simulink library "PortLib"  (Simulink 7.6)
settings: Solver=ode45  StartTime=0.0  StopTime=10.0  RelTol=1e-3
libraries: orocos_taskcontext x31, simulink x22
settings Model: Creator=Haus  LastModifiedBy=sendobry

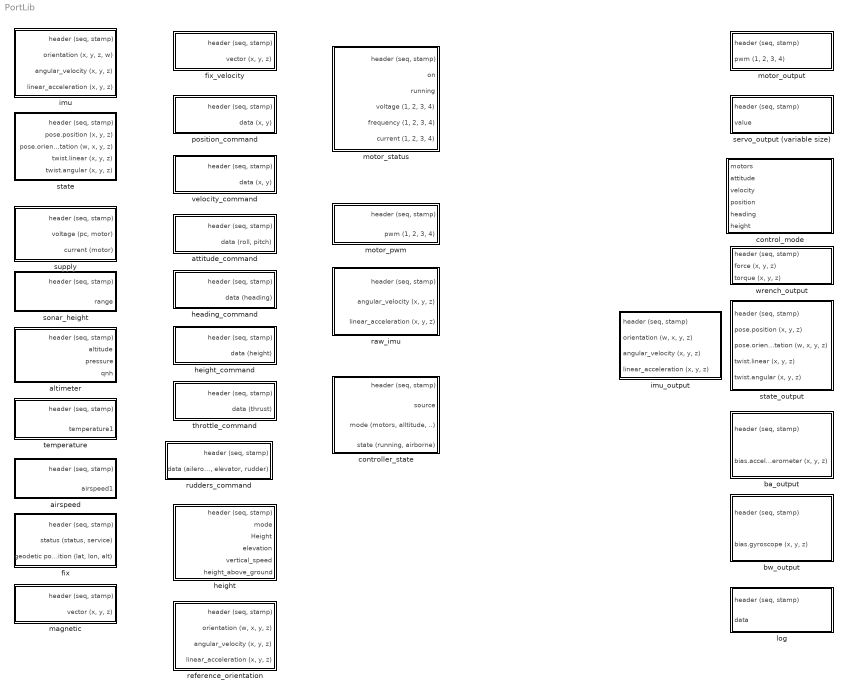
== system PortLib ==
  airspeed : Subsystem
  altimeter : Subsystem
  attitude_command : Subsystem
  ba_output : Subsystem
  bw_output : Subsystem
  control_mode : Subsystem
  controller_state : Subsystem
  fix : Subsystem
  fix_velocity : Subsystem
  heading_command : Subsystem
  height : Subsystem
  height_command : Subsystem
  imu : Subsystem
  imu_output : Subsystem
  log : Subsystem
  magnetic : Subsystem
  motor_output : Subsystem
  motor_pwm : Subsystem
  motor_status : Subsystem
  position_command : Subsystem
  raw_imu : Subsystem
  reference_orientation : Subsystem
  rudders_command : Subsystem
  servo_output (variable size) : Subsystem
  sonar_height : Subsystem
  state : Subsystem
  state_output : Subsystem
  supply : Subsystem
  temperature : Subsystem
  throttle_command : Subsystem
  velocity_command : Subsystem  AncestorBlock=PortLib/PositionXYCommand
  wrench_output : Subsystem

== system PortLib/airspeed ==
  Selector : Selector  IndexMode=Zero-based  InputPortWidth=3  IndexOptions=Index vector (dialog)  Indices=[0 1]  OutputSizes=1
  Selector1 : Selector  IndexMode=Zero-based  InputPortWidth=3  IndexOptions=Index vector (dialog)  Indices=[2]  OutputSizes=1
  airspeed : orocos_taskcontext/InputPort<array>  dpdesc=Port's Description  dpvalue=zeros(1,3)
      settings: AttributesFormatString=Value=%<dpvalue>
  "header (seq, stamp)" : Outport
  airspeed1 : Outport  Port=2
  wires:
  Selector/1 -> "header (seq, stamp)"/1
  airspeed/1 -> Selector1/1, Selector/1
  Selector1/1 -> airspeed1/1

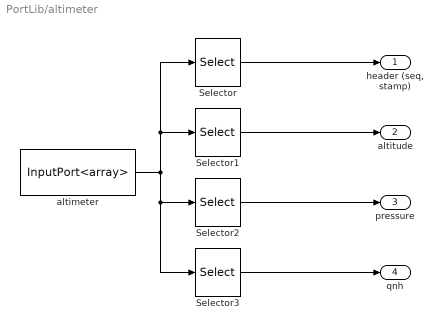
== system PortLib/altimeter ==
  Selector : Selector  IndexMode=Zero-based  InputPortWidth=5  IndexOptions=Index vector (dialog)  Indices=[0 1]  OutputSizes=1
  Selector1 : Selector  IndexMode=Zero-based  InputPortWidth=5  IndexOptions=Index vector (dialog)  Indices=[2]  OutputSizes=1
  Selector2 : Selector  IndexMode=Zero-based  InputPortWidth=5  IndexOptions=Index vector (dialog)  Indices=[3]  OutputSizes=1
  Selector3 : Selector  IndexMode=Zero-based  InputPortWidth=5  IndexOptions=Index vector (dialog)  Indices=[4]  OutputSizes=1
  altimeter : orocos_taskcontext/InputPort<array>  dpdesc=Port's Description  dpvalue=zeros(1,5)
      settings: AttributesFormatString=Value=%<dpvalue>
  "header (seq, stamp)" : Outport
  altitude : Outport  Port=2
  pressure : Outport  Port=3
  qnh : Outport  Port=4
  wires:
  Selector/1 -> "header (seq, stamp)"/1
  altimeter/1 -> Selector1/1, Selector/1, Selector2/1, Selector3/1
  Selector2/1 -> pressure/1
  Selector1/1 -> altitude/1
  Selector3/1 -> qnh/1

== system PortLib/attitude_command ==
  Selector : Selector  IndexMode=Zero-based  InputPortWidth=4  IndexOptions=Index vector (dialog)  Indices=[0 1]  OutputSizes=1
  Selector1 : Selector  IndexMode=Zero-based  InputPortWidth=4  IndexOptions=Index vector (dialog)  Indices=[2 3]  OutputSizes=1
  attitude_command : orocos_taskcontext/InputPort<array>  dpdesc=Port's Description  dpvalue=zeros(1,4)
      settings: AttributesFormatString=Value=%<dpvalue>
  "header (seq, stamp)" : Outport
  "data (roll, pitch)" : Outport  Port=2
  wires:
  Selector/1 -> "header (seq, stamp)"/1
  attitude_command/1 -> Selector1/1, Selector/1
  Selector1/1 -> "data (roll, pitch)"/1

== system PortLib/ba_output ==
  "header (seq, stamp)" : Inport
  "bias.accelerometer (x, y, z)" : Inport  Port=2
  Mux1 : Mux  Inputs=2
  linear_acceleration_bias : orocos_taskcontext/OutputPort<array>  dpdesc=Port's Description  dpvalue=zeros(1,5)
      settings: AttributesFormatString=Value=%<dpvalue>
  wires:
  "header (seq, stamp)"/1 -> Mux1/1
  "bias.accelerometer (x, y, z)"/1 -> Mux1/2
  Mux1/1 -> linear_acceleration_bias/1

== system PortLib/bw_output ==
  "header (seq, stamp)" : Inport
  "bias.gyroscope (x, y, z)" : Inport  Port=2
  Mux1 : Mux  Inputs=2
  angular_velocity_bias : orocos_taskcontext/OutputPort<array>  dpdesc=Port's Description  dpvalue=zeros(1,5)
      settings: AttributesFormatString=Value=%<dpvalue>
  wires:
  Mux1/1 -> angular_velocity_bias/1
  "bias.gyroscope (x, y, z)"/1 -> Mux1/2
  "header (seq, stamp)"/1 -> Mux1/1

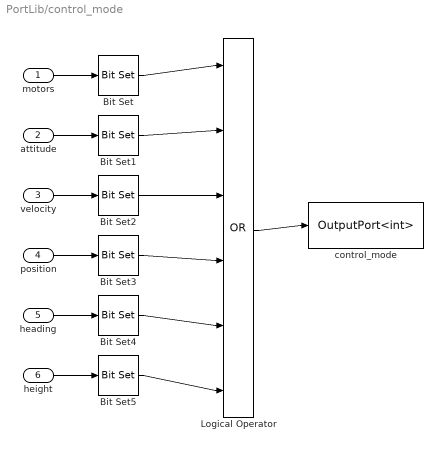
== system PortLib/control_mode ==
  motors : Inport
  attitude : Inport  Port=2
  velocity : Inport  Port=3
  position : Inport  Port=4
  heading : Inport  Port=5
  height : Inport  Port=6
  Bit Set : simulink/Logic and Bit Operations/Bit Set  iBit=0
  Bit Set1 : simulink/Logic and Bit Operations/Bit Set  iBit=1
  Bit Set2 : simulink/Logic and Bit Operations/Bit Set  iBit=2
  Bit Set3 : simulink/Logic and Bit Operations/Bit Set  iBit=3
  Bit Set4 : simulink/Logic and Bit Operations/Bit Set  iBit=4
  Bit Set5 : simulink/Logic and Bit Operations/Bit Set  iBit=5
  Logical Operator : Logic  Operator=OR  Inputs=6  AllPortsSameDT=off  OutDataTypeStr=boolean
  control_mode : orocos_taskcontext/OutputPort<int>  dpdesc=Port's Description  dpvalue=int32(0)
      settings: AttributesFormatString=Value=%<dpvalue>
  wires:
  Logical Operator/1 -> control_mode/1
  motors/1 -> Bit Set/1
  Bit Set/1 -> Logical Operator/1
  Bit Set1/1 -> Logical Operator/2
  Bit Set2/1 -> Logical Operator/3
  Bit Set3/1 -> Logical Operator/4
  Bit Set4/1 -> Logical Operator/5
  heading/1 -> Bit Set4/1
  position/1 -> Bit Set3/1
  velocity/1 -> Bit Set2/1
  attitude/1 -> Bit Set1/1
  height/1 -> Bit Set5/1
  Bit Set5/1 -> Logical Operator/6

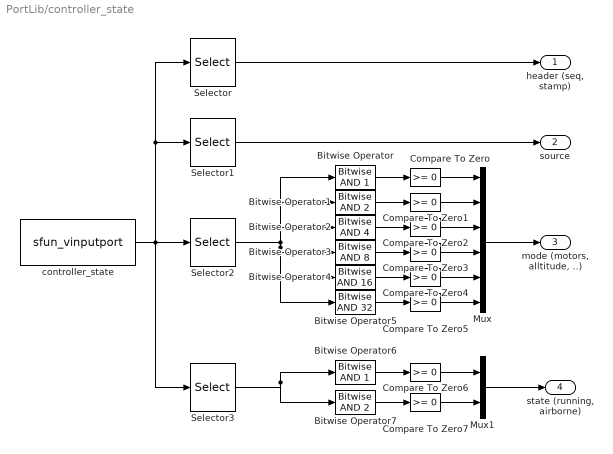
== system PortLib/controller_state ==
  Bitwise Operator : simulink/Logic and Bit Operations/Bitwise Operator  logicop=AND  UseBitMask=on  BitMask=1  BitMaskRealWorld=Stored Integer
  Bitwise Operator1 : simulink/Logic and Bit Operations/Bitwise Operator  logicop=AND  UseBitMask=on  BitMask=2  BitMaskRealWorld=Stored Integer
  Bitwise Operator2 : simulink/Logic and Bit Operations/Bitwise Operator  logicop=AND  UseBitMask=on  BitMask=4  BitMaskRealWorld=Stored Integer
  Bitwise Operator3 : simulink/Logic and Bit Operations/Bitwise Operator  logicop=AND  UseBitMask=on  BitMask=8  BitMaskRealWorld=Stored Integer
  Bitwise Operator4 : simulink/Logic and Bit Operations/Bitwise Operator  logicop=AND  UseBitMask=on  BitMask=16  BitMaskRealWorld=Stored Integer
  Bitwise Operator5 : simulink/Logic and Bit Operations/Bitwise Operator  logicop=AND  UseBitMask=on  BitMask=32  BitMaskRealWorld=Stored Integer
  Bitwise Operator6 : simulink/Logic and Bit Operations/Bitwise Operator  logicop=AND  UseBitMask=on  BitMask=1  BitMaskRealWorld=Stored Integer
  Bitwise Operator7 : simulink/Logic and Bit Operations/Bitwise Operator  logicop=AND  UseBitMask=on  BitMask=2  BitMaskRealWorld=Stored Integer
  Compare To Zero{,1..7} (8 alike) : simulink/Logic and Bit Operations/Compare To Zero  relop=>=  OutDataTypeStr=boolean
  Mux : Mux  Inputs=6
  Mux1 : Mux  Inputs=2
  Selector : Selector  IndexMode=Zero-based  InputPortWidth=5  IndexOptions=Index vector (dialog)  Indices=[0 1]  OutputSizes=1
  Selector1 : Selector  IndexMode=Zero-based  InputPortWidth=5  IndexOptions=Index vector (dialog)  Indices=2  OutputSizes=1
  Selector2 : Selector  IndexMode=Zero-based  InputPortWidth=5  IndexOptions=Index vector (dialog)  Indices=3  OutputSizes=1
  Selector3 : Selector  IndexMode=Zero-based  InputPortWidth=5  IndexOptions=Index vector (dialog)  Indices=4  OutputSizes=1
  controller_state : S-Function  FunctionName=sfun_vinputport  Parameters=dpdesc,dpvalue  EnableBusSupport=off  mask(DataPort<array>){dpdesc=Port's Description, dpvalue=zeros(1,5)}
      mask prompts: dpdesc "Description"; dpvalue "Initial Value (array)"
      mask help: A TaskContext's Vector DataPort holds a name, a description and an array of reals. It is used for inter-component data exchange. It translates to the C++ class RTT::DataPort< std::vector<double> >.
      settings: AttributesFormatString=Value=%<dpvalue>
      mask Display: fprintf('InputPort<array>')
  "header (seq, stamp)" : Outport
  source : Outport  Port=2
  "mode (motors, alltitude, ..)" : Outport  Port=3
  "state (running, airborne)" : Outport  Port=4
  wires:
  Selector/1 -> "header (seq, stamp)"/1
  Selector1/1 -> source/1
  Mux1/1 -> "state (running, airborne)"/1
  Mux/1 -> "mode (motors, alltitude, ..)"/1
  controller_state/1 -> Selector2/1, Selector3/1, Selector/1, Selector1/1
  Compare To Zero/1 -> Mux/1
  Bitwise Operator/1 -> Compare To Zero/1
  Bitwise Operator1/1 -> Compare To Zero1/1
  Bitwise Operator2/1 -> Compare To Zero2/1
  Bitwise Operator3/1 -> Compare To Zero3/1
  Bitwise Operator4/1 -> Compare To Zero4/1
  Bitwise Operator5/1 -> Compare To Zero5/1
  Compare To Zero1/1 -> Mux/2
  Compare To Zero2/1 -> Mux/3
  Compare To Zero3/1 -> Mux/4
  Compare To Zero4/1 -> Mux/5
  Compare To Zero5/1 -> Mux/6
  Selector2/1 -> Bitwise Operator/1, Bitwise Operator1/1, Bitwise Operator2/1, Bitwise Operator3/1, Bitwise Operator4/1, Bitwise Operator5/1
  Compare To Zero6/1 -> Mux1/1
  Bitwise Operator6/1 -> Compare To Zero6/1
  Bitwise Operator7/1 -> Compare To Zero7/1
  Compare To Zero7/1 -> Mux1/2
  Selector3/1 -> Bitwise Operator6/1, Bitwise Operator7/1

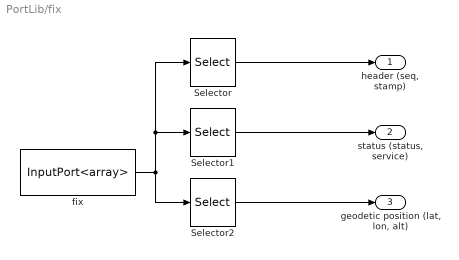
== system PortLib/fix ==
  Selector : Selector  IndexMode=Zero-based  InputPortWidth=7  IndexOptions=Index vector (dialog)  Indices=[0 1]  OutputSizes=1
  Selector1 : Selector  IndexMode=Zero-based  InputPortWidth=7  IndexOptions=Index vector (dialog)  Indices=[2 3]  OutputSizes=1
  Selector2 : Selector  IndexMode=Zero-based  InputPortWidth=7  IndexOptions=Index vector (dialog)  Indices=[4, 5, 6]  OutputSizes=1
  fix : orocos_taskcontext/InputPort<array>  dpdesc=Port's Description  dpvalue=zeros(1,7)
      settings: AttributesFormatString=Value=%<dpvalue>
  "header (seq, stamp)" : Outport
  "status (status, service)" : Outport  Port=2
  "geodetic position (lat, lon, alt)" : Outport  Port=3
  wires:
  Selector/1 -> "header (seq, stamp)"/1
  fix/1 -> Selector2/1, Selector1/1, Selector/1
  Selector2/1 -> "geodetic position (lat, lon, alt)"/1
  Selector1/1 -> "status (status, service)"/1

== system PortLib/fix_velocity ==
  Selector : Selector  IndexMode=Zero-based  InputPortWidth=5  IndexOptions=Index vector (dialog)  Indices=[0 1]  OutputSizes=1
  Selector1 : Selector  IndexMode=Zero-based  InputPortWidth=5  IndexOptions=Index vector (dialog)  Indices=[2 3 4]  OutputSizes=1
  fix_velocity : orocos_taskcontext/InputPort<array>  dpdesc=Port's Description  dpvalue=zeros(1,5)
      settings: AttributesFormatString=Value=%<dpvalue>
  "header (seq, stamp)" : Outport
  "vector (x, y, z)" : Outport  Port=2
  wires:
  Selector1/1 -> "vector (x, y, z)"/1
  fix_velocity/1 -> Selector/1, Selector1/1
  Selector/1 -> "header (seq, stamp)"/1

== system PortLib/heading_command ==
  Selector : Selector  IndexMode=Zero-based  InputPortWidth=3  IndexOptions=Index vector (dialog)  Indices=[0 1]  OutputSizes=1
  Selector1 : Selector  IndexMode=Zero-based  InputPortWidth=3  IndexOptions=Index vector (dialog)  Indices=[2]  OutputSizes=1
  heading_command : orocos_taskcontext/InputPort<array>  dpdesc=Port's Description  dpvalue=zeros(1,3)
      settings: AttributesFormatString=Value=%<dpvalue>
  "header (seq, stamp)" : Outport
  data (heading) : Outport  Port=2
  wires:
  Selector1/1 -> data (heading)/1
  heading_command/1 -> Selector/1, Selector1/1
  Selector/1 -> "header (seq, stamp)"/1

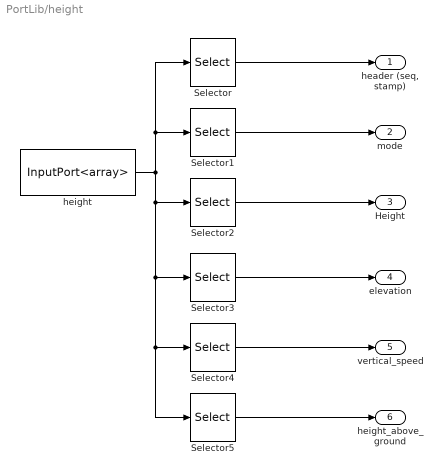
== system PortLib/height ==
  Selector : Selector  IndexMode=Zero-based  InputPortWidth=7  IndexOptions=Index vector (dialog)  Indices=[0 1]  OutputSizes=1
  Selector1 : Selector  IndexMode=Zero-based  InputPortWidth=7  IndexOptions=Index vector (dialog)  Indices=[2]  OutputSizes=1
  Selector2 : Selector  IndexMode=Zero-based  InputPortWidth=7  IndexOptions=Index vector (dialog)  Indices=[3]  OutputSizes=1
  Selector3 : Selector  IndexMode=Zero-based  InputPortWidth=7  IndexOptions=Index vector (dialog)  Indices=[4]  OutputSizes=1
  Selector4 : Selector  IndexMode=Zero-based  InputPortWidth=7  IndexOptions=Index vector (dialog)  Indices=[5]  OutputSizes=1
  Selector5 : Selector  IndexMode=Zero-based  InputPortWidth=7  IndexOptions=Index vector (dialog)  Indices=[6]  OutputSizes=1
  height : orocos_taskcontext/InputPort<array>  dpdesc=Port's Description  dpvalue=zeros(1,7)
      settings: AttributesFormatString=Value=%<dpvalue>
  "header (seq, stamp)" : Outport
  mode : Outport  Port=2
  Height : Outport  Port=3
  elevation : Outport  Port=4
  vertical_speed : Outport  Port=5
  height_above_ground : Outport  Port=6
  wires:
  Selector1/1 -> mode/1
  Selector2/1 -> Height/1
  height/1 -> Selector/1, Selector1/1, Selector2/1, Selector3/1, Selector4/1, Selector5/1
  Selector/1 -> "header (seq, stamp)"/1
  Selector3/1 -> elevation/1
  Selector4/1 -> vertical_speed/1
  Selector5/1 -> height_above_ground/1

== system PortLib/height_command ==
  Selector : Selector  IndexMode=Zero-based  InputPortWidth=3  IndexOptions=Index vector (dialog)  Indices=[0 1]  OutputSizes=1
  Selector1 : Selector  IndexMode=Zero-based  InputPortWidth=3  IndexOptions=Index vector (dialog)  Indices=[2]  OutputSizes=1
  height_command : orocos_taskcontext/InputPort<array>  dpdesc=Port's Description  dpvalue=zeros(1,3)
      settings: AttributesFormatString=Value=%<dpvalue>
  "header (seq, stamp)" : Outport
  data (height) : Outport  Port=2
  wires:
  Selector/1 -> "header (seq, stamp)"/1
  height_command/1 -> Selector1/1, Selector/1
  Selector1/1 -> data (height)/1

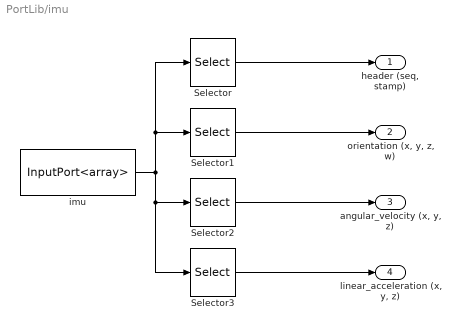
== system PortLib/imu ==
  Selector : Selector  IndexMode=Zero-based  InputPortWidth=12  IndexOptions=Index vector (dialog)  Indices=[0 1]  OutputSizes=1
  Selector1 : Selector  IndexMode=Zero-based  InputPortWidth=12  IndexOptions=Index vector (dialog)  Indices=[2 3 4 5]  OutputSizes=1
  Selector2 : Selector  IndexMode=Zero-based  InputPortWidth=12  IndexOptions=Index vector (dialog)  Indices=[6 7 8]  OutputSizes=1
  Selector3 : Selector  IndexMode=Zero-based  InputPortWidth=12  IndexOptions=Index vector (dialog)  Indices=[9 10 11]  OutputSizes=1
  imu : orocos_taskcontext/InputPort<array>  dpdesc=Port's Description  dpvalue=zeros(1,12)
      settings: AttributesFormatString=Value=%<dpvalue>
  "header (seq, stamp)" : Outport
  "orientation (x, y, z, w)" : Outport  Port=2
  "angular_velocity (x, y, z)" : Outport  Port=3
  "linear_acceleration (x, y, z)" : Outport  Port=4
  wires:
  Selector1/1 -> "orientation (x, y, z, w)"/1
  Selector2/1 -> "angular_velocity (x, y, z)"/1
  Selector3/1 -> "linear_acceleration (x, y, z)"/1
  imu/1 -> Selector/1, Selector1/1, Selector2/1, Selector3/1
  Selector/1 -> "header (seq, stamp)"/1

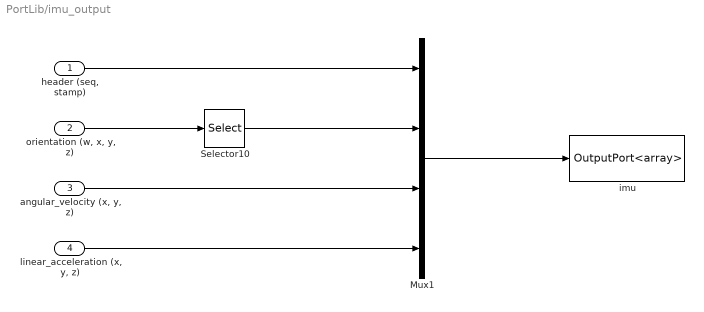
== system PortLib/imu_output ==
  "header (seq, stamp)" : Inport
  "orientation (w, x, y, z)" : Inport  Port=2
  "angular_velocity (x, y, z)" : Inport  Port=3
  "linear_acceleration (x, y, z)" : Inport  Port=4
  Mux1 : Mux
  Selector10 : Selector  InputPortWidth=4  IndexOptions=Index vector (dialog)  Indices=[2 3 4 1]  OutputSizes=1
  imu : orocos_taskcontext/OutputPort<array>  dpdesc=Port's Description  dpvalue=zeros(1,12)
      settings: AttributesFormatString=Value=%<dpvalue>
  wires:
  Mux1/1 -> imu/1
  "header (seq, stamp)"/1 -> Mux1/1
  "orientation (w, x, y, z)"/1 -> Selector10/1
  "angular_velocity (x, y, z)"/1 -> Mux1/3
  "linear_acceleration (x, y, z)"/1 -> Mux1/4
  Selector10/1 -> Mux1/2

== system PortLib/log ==
  "header (seq, stamp)" : Inport
  data : Inport  Port=2
  Mux1 : Mux  Inputs=2
  log : orocos_taskcontext/OutputPort<array>  dpdesc=Port's Description  dpvalue=zeros(1,2)
      settings: AttributesFormatString=Value=%<dpvalue>
  wires:
  Mux1/1 -> log/1
  data/1 -> Mux1/2
  "header (seq, stamp)"/1 -> Mux1/1

== system PortLib/magnetic ==
  Selector : Selector  IndexMode=Zero-based  InputPortWidth=5  IndexOptions=Index vector (dialog)  Indices=[0 1]  OutputSizes=1
  Selector1 : Selector  IndexMode=Zero-based  InputPortWidth=5  IndexOptions=Index vector (dialog)  Indices=[2 3 4]  OutputSizes=1
  magnetic : orocos_taskcontext/InputPort<array>  dpdesc=Port's Description  dpvalue=zeros(1,5)
      settings: AttributesFormatString=Value=%<dpvalue>
  "header (seq, stamp)" : Outport
  "vector (x, y, z)" : Outport  Port=2
  wires:
  Selector/1 -> "header (seq, stamp)"/1
  magnetic/1 -> Selector1/1, Selector/1
  Selector1/1 -> "vector (x, y, z)"/1

== system PortLib/motor_output ==
  "header (seq, stamp)" : Inport
  "pwm (1, 2, 3, 4)" : Inport  Port=2
  Mux1 : Mux  Inputs=2
  motor_output : orocos_taskcontext/OutputPort<array>  dpdesc=Port's Description  dpvalue=zeros(1,6)
      settings: AttributesFormatString=Value=%<dpvalue>
  wires:
  "header (seq, stamp)"/1 -> Mux1/1
  "pwm (1, 2, 3, 4)"/1 -> Mux1/2
  Mux1/1 -> motor_output/1

== system PortLib/motor_pwm ==
  Selector : Selector  IndexMode=Zero-based  InputPortWidth=6  IndexOptions=Index vector (dialog)  Indices=[0 1]  OutputSizes=1
  Selector1 : Selector  IndexMode=Zero-based  InputPortWidth=6  IndexOptions=Index vector (dialog)  Indices=[2:5]  OutputSizes=1
  motor_pwm : orocos_taskcontext/InputPort<array>  dpdesc=Port's Description  dpvalue=zeros(1,6)
      settings: AttributesFormatString=Value=%<dpvalue>
  "header (seq, stamp)" : Outport
  "pwm (1, 2, 3, 4)" : Outport  Port=2
  wires:
  Selector/1 -> "header (seq, stamp)"/1
  motor_pwm/1 -> Selector/1, Selector1/1
  Selector1/1 -> "pwm (1, 2, 3, 4)"/1

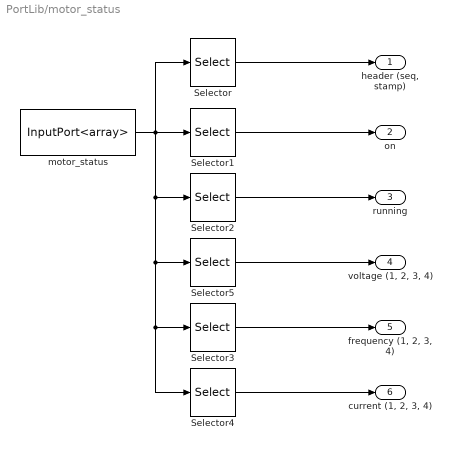
== system PortLib/motor_status ==
  Selector : Selector  IndexMode=Zero-based  InputPortWidth=16  IndexOptions=Index vector (dialog)  Indices=[0 1]  OutputSizes=1
  Selector1 : Selector  IndexMode=Zero-based  InputPortWidth=16  IndexOptions=Index vector (dialog)  Indices=[2]  OutputSizes=1
  Selector2 : Selector  IndexMode=Zero-based  InputPortWidth=16  IndexOptions=Index vector (dialog)  Indices=3  OutputSizes=1
  Selector3 : Selector  IndexMode=Zero-based  InputPortWidth=16  IndexOptions=Index vector (dialog)  Indices=[8:11]  OutputSizes=1
  Selector4 : Selector  IndexMode=Zero-based  InputPortWidth=16  IndexOptions=Index vector (dialog)  Indices=[12:15]  OutputSizes=1
  Selector5 : Selector  IndexMode=Zero-based  InputPortWidth=16  IndexOptions=Index vector (dialog)  Indices=[4:7]  OutputSizes=1
  motor_status : orocos_taskcontext/InputPort<array>  dpdesc=Port's Description  dpvalue=zeros(1,12)
      settings: AttributesFormatString=Value=%<dpvalue>
  "header (seq, stamp)" : Outport
  on : Outport  Port=2
  running : Outport  Port=3
  "voltage (1, 2, 3, 4)" : Outport  Port=4
  "frequency (1, 2, 3, 4)" : Outport  Port=5
  "current (1, 2, 3, 4)" : Outport  Port=6
  wires:
  motor_status/1 -> Selector/1, Selector1/1, Selector2/1, Selector5/1, Selector3/1, Selector4/1
  Selector/1 -> "header (seq, stamp)"/1
  Selector1/1 -> on/1
  Selector2/1 -> running/1
  Selector3/1 -> "frequency (1, 2, 3, 4)"/1
  Selector4/1 -> "current (1, 2, 3, 4)"/1
  Selector5/1 -> "voltage (1, 2, 3, 4)"/1

== system PortLib/position_command ==
  Selector : Selector  IndexMode=Zero-based  InputPortWidth=4  IndexOptions=Index vector (dialog)  Indices=[0 1]  OutputSizes=1
  Selector1 : Selector  IndexMode=Zero-based  InputPortWidth=4  IndexOptions=Index vector (dialog)  Indices=[2 3]  OutputSizes=1
  position_command : orocos_taskcontext/InputPort<array>  dpdesc=Port's Description  dpvalue=zeros(1,4)
      settings: AttributesFormatString=Value=%<dpvalue>
  "header (seq, stamp)" : Outport
  "data (x, y)" : Outport  Port=2
  wires:
  Selector/1 -> "header (seq, stamp)"/1
  position_command/1 -> Selector1/1, Selector/1
  Selector1/1 -> "data (x, y)"/1

== system PortLib/raw_imu ==
  Selector : Selector  IndexMode=Zero-based  InputPortWidth=12  IndexOptions=Index vector (dialog)  Indices=[0 1]  OutputSizes=1
  Selector2 : Selector  IndexMode=Zero-based  InputPortWidth=12  IndexOptions=Index vector (dialog)  Indices=[6 7 8]  OutputSizes=1
  Selector3 : Selector  IndexMode=Zero-based  InputPortWidth=12  IndexOptions=Index vector (dialog)  Indices=[9 10 11]  OutputSizes=1
  raw_imu : orocos_taskcontext/InputPort<array>  dpdesc=Port's Description  dpvalue=zeros(1,12)
      settings: AttributesFormatString=Value=%<dpvalue>
  "header (seq, stamp)" : Outport
  "angular_velocity (x, y, z)" : Outport  Port=2
  "linear_acceleration (x, y, z)" : Outport  Port=3
  wires:
  Selector/1 -> "header (seq, stamp)"/1
  raw_imu/1 -> Selector3/1, Selector2/1, Selector/1
  Selector3/1 -> "linear_acceleration (x, y, z)"/1
  Selector2/1 -> "angular_velocity (x, y, z)"/1

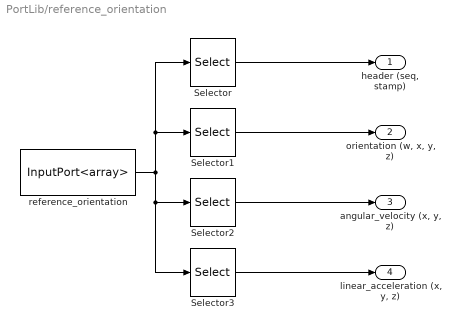
== system PortLib/reference_orientation ==
  Selector : Selector  IndexMode=Zero-based  InputPortWidth=12  IndexOptions=Index vector (dialog)  Indices=[0 1]  OutputSizes=1
  Selector1 : Selector  IndexMode=Zero-based  InputPortWidth=12  IndexOptions=Index vector (dialog)  Indices=[5 2 3 4]  OutputSizes=1
  Selector2 : Selector  IndexMode=Zero-based  InputPortWidth=12  IndexOptions=Index vector (dialog)  Indices=[6 7 8]  OutputSizes=1
  Selector3 : Selector  IndexMode=Zero-based  InputPortWidth=12  IndexOptions=Index vector (dialog)  Indices=[9 10 11]  OutputSizes=1
  reference_orientation : orocos_taskcontext/InputPort<array>  dpdesc=Port's Description  dpvalue=zeros(1,12)
      settings: AttributesFormatString=Value=%<dpvalue>
  "header (seq, stamp)" : Outport
  "orientation (w, x, y, z)" : Outport  Port=2
  "angular_velocity (x, y, z)" : Outport  Port=3
  "linear_acceleration (x, y, z)" : Outport  Port=4
  wires:
  Selector/1 -> "header (seq, stamp)"/1
  reference_orientation/1 -> Selector3/1, Selector2/1, Selector1/1, Selector/1
  Selector3/1 -> "linear_acceleration (x, y, z)"/1
  Selector2/1 -> "angular_velocity (x, y, z)"/1
  Selector1/1 -> "orientation (w, x, y, z)"/1

== system PortLib/rudders_command ==
  Selector : Selector  IndexMode=Zero-based  InputPortWidth=5  IndexOptions=Index vector (dialog)  Indices=[0 1]  OutputSizes=1
  Selector1 : Selector  IndexMode=Zero-based  InputPortWidth=5  IndexOptions=Index vector (dialog)  Indices=[2 3 4]  OutputSizes=1
  rudders_command : orocos_taskcontext/InputPort<array>  dpdesc=Port's Description  dpvalue=zeros(1,5)
      settings: AttributesFormatString=Value=%<dpvalue>
  "header (seq, stamp)" : Outport
  "data (aileron, elevator, rudder)" : Outport  Port=2
  wires:
  Selector1/1 -> "data (aileron, elevator, rudder)"/1
  rudders_command/1 -> Selector/1, Selector1/1
  Selector/1 -> "header (seq, stamp)"/1

== system PortLib/servo_output (variable size) ==
  "header (seq, stamp)" : Inport
  value : Inport  Port=2
  Mux1 : Mux  Inputs=2
  servo_output : orocos_taskcontext/OutputPort<array>  dpdesc=Port's Description  dpvalue=zeros(1,6)
      settings: AttributesFormatString=Value=%<dpvalue>
  wires:
  Mux1/1 -> servo_output/1
  value/1 -> Mux1/2
  "header (seq, stamp)"/1 -> Mux1/1

== system PortLib/sonar_height ==
  Selector : Selector  IndexMode=Zero-based  InputPortWidth=3  IndexOptions=Index vector (dialog)  Indices=[0 1]  OutputSizes=1
  Selector1 : Selector  IndexMode=Zero-based  InputPortWidth=3  IndexOptions=Index vector (dialog)  Indices=[2]  OutputSizes=1
  sonar_height : orocos_taskcontext/InputPort<array>  dpdesc=Port's Description  dpvalue=zeros(1,3)
      settings: AttributesFormatString=Value=%<dpvalue>
  "header (seq, stamp)" : Outport
  range : Outport  Port=2
  wires:
  Selector/1 -> "header (seq, stamp)"/1
  sonar_height/1 -> Selector1/1, Selector/1
  Selector1/1 -> range/1

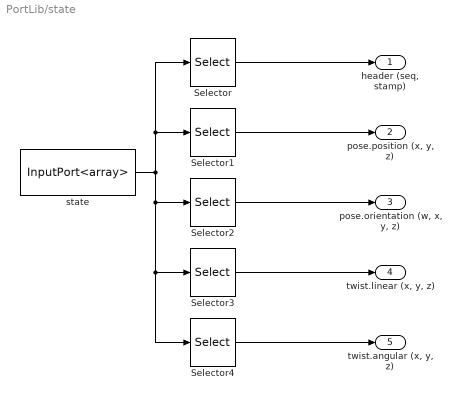
== system PortLib/state ==
  Selector : Selector  IndexMode=Zero-based  InputPortWidth=15  IndexOptions=Index vector (dialog)  Indices=[0 1]  OutputSizes=1
  Selector1 : Selector  IndexMode=Zero-based  InputPortWidth=15  IndexOptions=Index vector (dialog)  Indices=[2 3 4]  OutputSizes=1
  Selector2 : Selector  IndexMode=Zero-based  InputPortWidth=15  IndexOptions=Index vector (dialog)  Indices=[8 5 6 7]  OutputSizes=1
  Selector3 : Selector  IndexMode=Zero-based  InputPortWidth=15  IndexOptions=Index vector (dialog)  Indices=[9 10 11]  OutputSizes=1
  Selector4 : Selector  IndexMode=Zero-based  InputPortWidth=15  IndexOptions=Index vector (dialog)  Indices=[12 13 14]  OutputSizes=1
  state : orocos_taskcontext/InputPort<array>  dpdesc=Port's Description  dpvalue=zeros(1,15)
      settings: AttributesFormatString=Value=%<dpvalue>
  "header (seq, stamp)" : Outport
  "pose.position (x, y, z)" : Outport  Port=2
  "pose.orientation (w, x, y, z)" : Outport  Port=3
  "twist.linear (x, y, z)" : Outport  Port=4
  "twist.angular (x, y, z)" : Outport  Port=5
  wires:
  Selector/1 -> "header (seq, stamp)"/1
  state/1 -> Selector2/1, Selector3/1, Selector4/1, Selector1/1, Selector/1
  Selector3/1 -> "twist.linear (x, y, z)"/1
  Selector2/1 -> "pose.orientation (w, x, y, z)"/1
  Selector1/1 -> "pose.position (x, y, z)"/1
  Selector4/1 -> "twist.angular (x, y, z)"/1

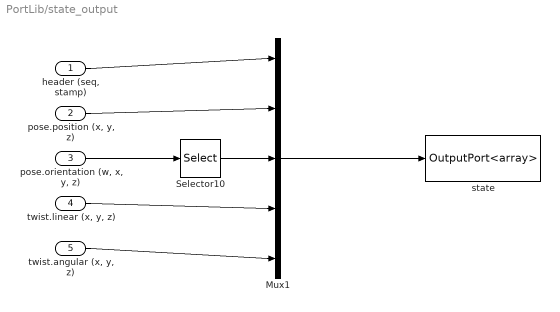
== system PortLib/state_output ==
  "header (seq, stamp)" : Inport
  "pose.position (x, y, z)" : Inport  Port=2
  "pose.orientation (w, x, y, z)" : Inport  Port=3
  "twist.linear (x, y, z)" : Inport  Port=4
  "twist.angular (x, y, z)" : Inport  Port=5
  Mux1 : Mux  Inputs=5
  Selector10 : Selector  InputPortWidth=4  IndexOptions=Index vector (dialog)  Indices=[2 3 4 1]  OutputSizes=1
  state : orocos_taskcontext/OutputPort<array>  dpdesc=Port's Description  dpvalue=zeros(1,15)
      settings: AttributesFormatString=Value=%<dpvalue>
  wires:
  Mux1/1 -> state/1
  "pose.position (x, y, z)"/1 -> Mux1/2
  "header (seq, stamp)"/1 -> Mux1/1
  "pose.orientation (w, x, y, z)"/1 -> Selector10/1
  "twist.linear (x, y, z)"/1 -> Mux1/4
  "twist.angular (x, y, z)"/1 -> Mux1/5
  Selector10/1 -> Mux1/3

== system PortLib/supply ==
  Selector : Selector  IndexMode=Zero-based  InputPortWidth=5  IndexOptions=Index vector (dialog)  Indices=[0 1]  OutputSizes=1
  Selector1 : Selector  IndexMode=Zero-based  InputPortWidth=5  IndexOptions=Index vector (dialog)  Indices=[2 3]  OutputSizes=1
  Selector2 : Selector  IndexMode=Zero-based  InputPortWidth=5  IndexOptions=Index vector (dialog)  Indices=[4]  OutputSizes=1
  supply : orocos_taskcontext/InputPort<array>  dpdesc=Port's Description  dpvalue=zeros(1,5)
      settings: AttributesFormatString=Value=%<dpvalue>
  "header (seq, stamp)" : Outport
  "voltage (pc, motor)" : Outport  Port=2
  current (motor) : Outport  Port=3
  wires:
  Selector1/1 -> "voltage (pc, motor)"/1
  Selector2/1 -> current (motor)/1
  supply/1 -> Selector/1, Selector1/1, Selector2/1
  Selector/1 -> "header (seq, stamp)"/1

== system PortLib/temperature ==
  Selector : Selector  IndexMode=Zero-based  InputPortWidth=3  IndexOptions=Index vector (dialog)  Indices=[0 1]  OutputSizes=1
  Selector1 : Selector  IndexMode=Zero-based  InputPortWidth=3  IndexOptions=Index vector (dialog)  Indices=[2]  OutputSizes=1
  temperature : orocos_taskcontext/InputPort<array>  dpdesc=Port's Description  dpvalue=zeros(1,3)
      settings: AttributesFormatString=Value=%<dpvalue>
  "header (seq, stamp)" : Outport
  temperature1 : Outport  Port=2
  wires:
  Selector1/1 -> temperature1/1
  temperature/1 -> Selector/1, Selector1/1
  Selector/1 -> "header (seq, stamp)"/1

== system PortLib/throttle_command ==
  Selector : Selector  IndexMode=Zero-based  InputPortWidth=3  IndexOptions=Index vector (dialog)  Indices=[0 1]  OutputSizes=1
  Selector1 : Selector  IndexMode=Zero-based  InputPortWidth=3  IndexOptions=Index vector (dialog)  Indices=[2]  OutputSizes=1
  throttle_command : orocos_taskcontext/InputPort<array>  dpdesc=Port's Description  dpvalue=zeros(1,3)
      settings: AttributesFormatString=Value=%<dpvalue>
  "header (seq, stamp)" : Outport
  data (thrust) : Outport  Port=2
  wires:
  Selector1/1 -> data (thrust)/1
  throttle_command/1 -> Selector/1, Selector1/1
  Selector/1 -> "header (seq, stamp)"/1

== system PortLib/velocity_command ==
  Selector : Selector  IndexMode=Zero-based  InputPortWidth=4  IndexOptions=Index vector (dialog)  Indices=[0 1]  OutputSizes=1
  Selector1 : Selector  IndexMode=Zero-based  InputPortWidth=4  IndexOptions=Index vector (dialog)  Indices=[2 3]  OutputSizes=1
  velocity_command : orocos_taskcontext/InputPort<array>  dpdesc=Port's Description  dpvalue=zeros(1,4)
      settings: AttributesFormatString=Value=%<dpvalue>
  "header (seq, stamp)" : Outport
  "data (x, y)" : Outport  Port=2
  wires:
  Selector1/1 -> "data (x, y)"/1
  velocity_command/1 -> Selector/1, Selector1/1
  Selector/1 -> "header (seq, stamp)"/1

== system PortLib/wrench_output ==
  "header (seq, stamp)" : Inport
  "force (x, y, z)" : Inport  Port=2
  "torque (x, y, z)" : Inport  Port=3
  Mux1 : Mux  Inputs=3
  wrench_output : orocos_taskcontext/OutputPort<array>  dpdesc=Port's Description  dpvalue=zeros(1,8)
      settings: AttributesFormatString=Value=%<dpvalue>
  wires:
  "header (seq, stamp)"/1 -> Mux1/1
  "force (x, y, z)"/1 -> Mux1/2
  Mux1/1 -> wrench_output/1
  "torque (x, y, z)"/1 -> Mux1/3
